simulink model "SistemaPF"  (R2024b)
settings: Solver=VariableStepAuto  StartTime=0.0  StopTime=10  RelTol=1e-3
libraries: slpidlib x1
settings Model: Creator=user
settings DataIOCC: TimeSaveName=t
settings DebuggingCC: UnconnectedInputMsg=warning  UnconnectedOutputMsg=warning  UnconnectedLineMsg=warning
settings ModelReferenceCC: EnableRefExpFcnMdlSchedulingChecks=on
settings RTWCC: GPUComputeCapability=3.5  DLArmComputeVersion=19.05

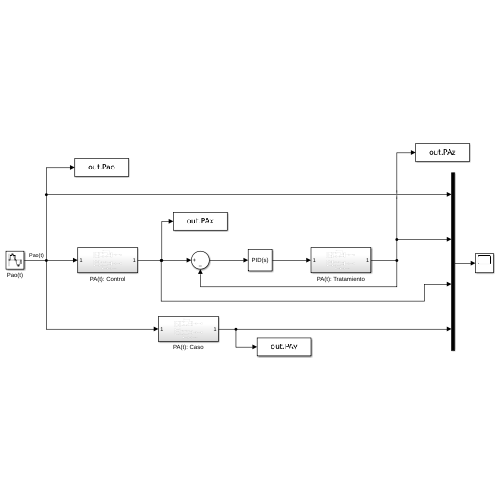
[thumbnail: Simulink's stored preview of the top-level diagram]
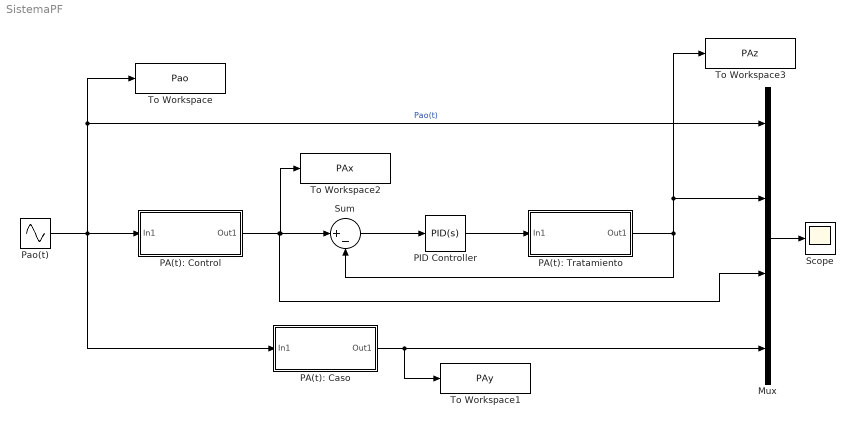
== system SistemaPF ==
  Mux : Mux
  PA(t): Caso : Subsystem
  PA(t): Control : Subsystem
  PA(t): Tratamiento : Subsystem
  PID Controller : slpidlib/PID Controller  Controller=PID  Form=Parallel  TimeDomain=Continuous-time  UseExternalTs=off  SampleTime=-1  IntegratorMethod=Forward Euler  FilterMethod=Forward Euler  ControllerParametersSource=internal  P=10.7123  I=13.7603  UseKiTs=off  D=1.4435  UseExternalDerivativeSource=off  N=651.125593180184  UseFilter=on  TunerSelectOption=Transfer Function Based (PID Tuner App)  InitialConditionSource=internal  InitialConditionForIntegrator=0  InitialConditionForFilter=0  DifferentiatorICPrevScaledInput=0  ExternalReset=none  TrackingMode=off  Kt=1  LimitOutput=off  SatLimitsSource=internal  UpperSaturationLimit=inf  LowerSaturationLimit=-inf  LinearizeAsGain=on  AntiWindupMode=none  Kb=1  LimitIntegrator=off  UpperIntegratorSaturationLimit=inf  LowerIntegratorSaturationLimit=-inf  POutMin=[]  POutMax=[]  IOutMin=[]  IOutMax=[]  DOutMin=[]  DOutMax=[]  NOutMin=[]  NOutMax=[]  SumOutMin=[]  SumOutMax=[]  SaturationOutMin=[]  SaturationOutMax=[]  PParamMin=[]  PParamMax=[]  IParamMin=[]  IParamMax=[]  DParamMin=[]  DParamMax=[]  NParamMin=[]  NParamMax=[]  KbParamMin=[]  KbParamMax=[]  KtParamMin=[]  KtParamMax=[]  KbOutMin=[]  KbOutMax=[]  KtOutMin=[]  KtOutMax=[]  IntegratorOutMin=[]  IntegratorOutMax=[]  FilterOutMin=[]  FilterOutMax=[]  SumI1OutMin=[]  SumI1OutMax=[]  SumI2OutMin=[]  SumI2OutMax=[]  SumI3OutMin=[]  SumI3OutMax=[]  SumI4OutMin=[]  SumI4OutMax=[]  SumDOutMin=[]  SumDOutMax=[]  DifferentiatorOutMin=[]  DifferentiatorOutMax=[]  FilterDiffOutCoefMin=[]  FilterDiffOutCoefMax=[]  ReciprocalOutMin=[]  ReciprocalOutMax=[]  SumDenOutMin=[]  SumDenOutMax=[]  SumNumOutMin=[]  SumNumOutMax=[]  DivideOutMin=[]  DivideOutMax=[]  UdiffTsProdOutMin=[]  UdiffTsProdOutMax=[]  NTsProdOutMin=[]  NTsProdOutMax=[]  UintegralTsProdOutMin=[]  UintegralTsProdOutMax=[]  UngainTsProdOutMin=[]  UngainTsProdOutMax=[]  ClampingZeroOutDataTypeStr=Inherit: Inherit via back propagation  ClampingZeroOutMin=[]  ClampingZeroOutMax=[]  FilterDenConstantOutDataTypeStr=Inherit: Inherit via back propagation  FilterDenConstantOutMin=[]  FilterDenConstantOutMax=[]  PCopyOutDataTypeStr=Inherit: Inherit via back propagation  PCopyOutMin=[]  PCopyOutMax=[]  NCopyOutDataTypeStr=Inherit: Inherit via back propagation  NCopyOutMin=[]  NCopyOutMax=[]  IntegratorContinuousStateAttributes=''  IntegratorStateMustResolveToSignalObject=off  IntegratorRTWStateStorageClass=Auto  FilterContinuousStateAttributes=''  FilterStateMustResolveToSignalObject=off  FilterRTWStateStorageClass=Auto  ParallelPVariant=InternalParameters  IdealPVariant=Disabled  IVariant=InternalParameters  DVariant=InternalParameters  IntegratorVariant=Continuous  SatVariant=Disabled  AWVariant=Passthrough  PCopyVariant=Disabled  TRVariant=Disabled  FdbkBlocksVariant=Forward  IdealPFdbkVariant=Disabled  SatFdbkVariant=Disabled  DerivativeFilterVariant=ContFilter  NVariant=InternalParameters  NCopyVariant=Disabled  FilterICVariant=InternalICsFilter  IntegratorICVariant=InternalICs  ExternalResetVariant=Disabled  TRSumVariant=Passthrough  SumFdbkVariant=Disabled  SumVariant=Sum_PID  TsampFilterVariant=InternalTs  TsampNgainVariant=Passthrough  TsampIntegralVariant=Disabled_SignalSpec  ExternalSaturationOutDataTypeStr=Inherit: Same as second input  DerivativeSourceVariant=ErrorSignal  PreIntVariant=InternalPreInt
  Pao(t) : Sin  Frequency=pi/2  SampleTime=0.001
  Scope : Scope
  Sum : Sum  Inputs=|+-
  To Workspace : ToWorkspace  VariableName=Pao  SampleTime=-1
  To Workspace1 : ToWorkspace  VariableName=PAy  SampleTime=-1
  To Workspace2 : ToWorkspace  VariableName=PAx  SampleTime=-1
  To Workspace3 : ToWorkspace  VariableName=PAz  SampleTime=-1
  wires:
  Sum/1 -> PID Controller/1
  Mux/1 -> Scope/1
  PA(t): Tratamiento/1(Out1) -> Sum/2, To Workspace3/1, Mux/2
  PA(t): Caso/1(Out1) -> To Workspace1/1, Mux/4
  PA(t): Control/1(Out1) -> Mux/3, To Workspace2/1, Sum/1
  PID Controller/1 -> PA(t): Tratamiento/1(In1)
  Pao(t)/1 -> PA(t): Caso/1(In1), To Workspace/1, Mux/1, PA(t): Control/1(In1)  "Pao(t)"

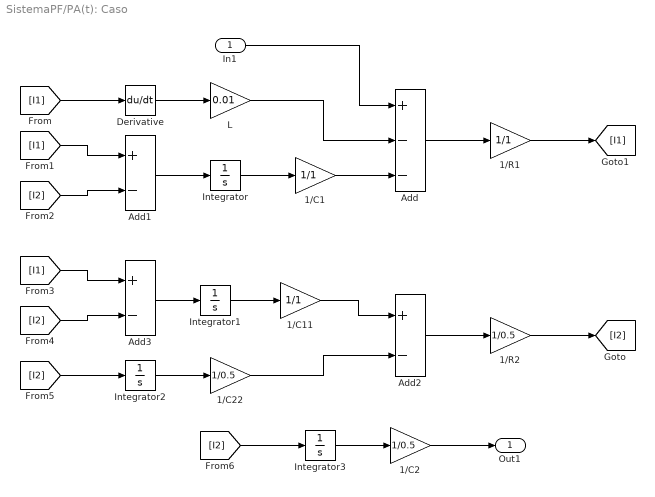
== system SistemaPF/PA(t): Caso ==
  In1 : Inport
  1/C1 : Gain  Gain=1/1
  1/C11 : Gain  Gain=1/1
  1/C2 : Gain  Gain=1/0.5
  1/C22 : Gain  Gain=1/0.5
  1/R1 : Gain  Gain=1/1
  1/R2 : Gain  Gain=1/0.5
  Add : Sum  Inputs=+--
  Add1 : Sum  Inputs=+-
  Add2 : Sum  Inputs=+-
  Add3 : Sum  Inputs=+-
  Derivative : Derivative
  Integrator{,1..3} (4 alike) : Integrator
  L : Gain  Gain=0.01
  Out1 : Outport
  wires:
  [I1] -> Derivative/1
  Derivative/1 -> L/1
  [I1] -> Add1/1
  [I2] -> Add1/2
  Add2/1 -> 1/R2/1
  1/R2/1 -> [I2]
  [I2] -> Add3/2
  [I1] -> Add3/1
  1/C11/1 -> Add2/1
  Add1/1 -> Integrator/1
  Integrator/1 -> 1/C1/1
  Add3/1 -> Integrator1/1
  Integrator1/1 -> 1/C11/1
  [I2] -> Integrator2/1
  Integrator2/1 -> 1/C22/1
  1/C22/1 -> Add2/2
  [I2] -> Integrator3/1
  Integrator3/1 -> 1/C2/1
  1/C2/1 -> Out1/1
  1/C1/1 -> Add/3
  L/1 -> Add/2
  In1/1 -> Add/1
  Add/1 -> 1/R1/1
  1/R1/1 -> [I1]

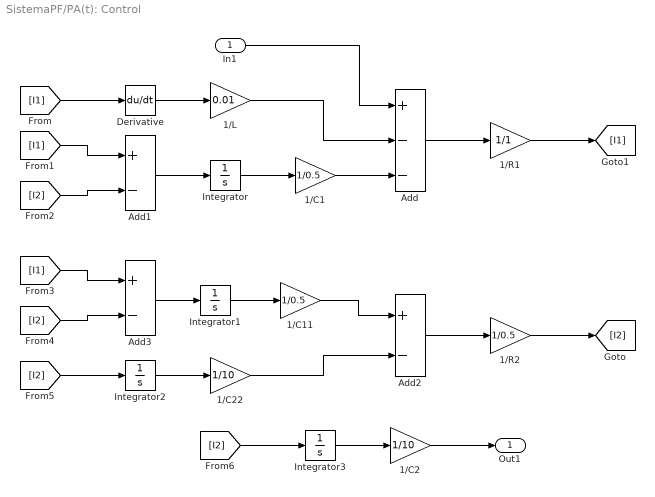
== system SistemaPF/PA(t): Control ==
  In1 : Inport
  1/C1 : Gain  Gain=1/0.5
  1/C11 : Gain  Gain=1/0.5
  1/C2 : Gain  Gain=1/10
  1/C22 : Gain  Gain=1/10
  1/L : Gain  Gain=0.01
  1/R1 : Gain  Gain=1/1
  1/R2 : Gain  Gain=1/0.5
  Add : Sum  Inputs=+--
  Add1 : Sum  Inputs=+-
  Add2 : Sum  Inputs=+-
  Add3 : Sum  Inputs=+-
  Derivative : Derivative
  Integrator{,1..3} (4 alike) : Integrator
  Out1 : Outport
  wires:
  [I1] -> Derivative/1
  Derivative/1 -> 1/L/1
  [I1] -> Add1/1
  [I2] -> Add1/2
  Add2/1 -> 1/R2/1
  1/R2/1 -> [I2]
  [I2] -> Add3/2
  [I1] -> Add3/1
  1/C11/1 -> Add2/1
  Add1/1 -> Integrator/1
  Integrator/1 -> 1/C1/1
  Add3/1 -> Integrator1/1
  Integrator1/1 -> 1/C11/1
  [I2] -> Integrator2/1
  Integrator2/1 -> 1/C22/1
  1/C22/1 -> Add2/2
  [I2] -> Integrator3/1
  Integrator3/1 -> 1/C2/1
  1/C2/1 -> Out1/1
  1/C1/1 -> Add/3
  1/L/1 -> Add/2
  In1/1 -> Add/1
  Add/1 -> 1/R1/1
  1/R1/1 -> [I1]

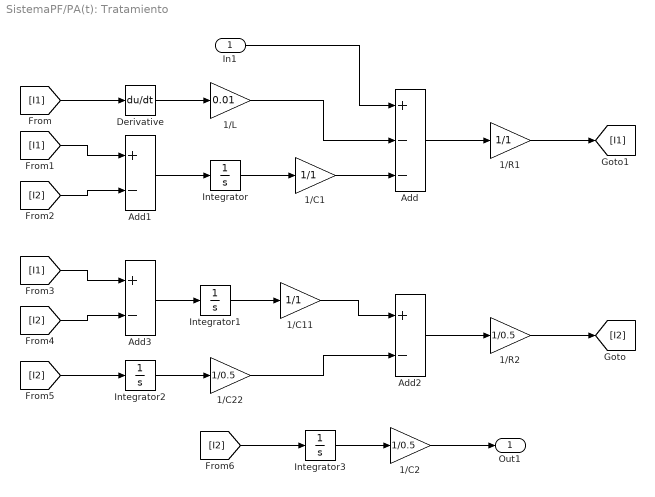
== system SistemaPF/PA(t): Tratamiento ==
  In1 : Inport
  1/C1 : Gain  Gain=1/1
  1/C11 : Gain  Gain=1/1
  1/C2 : Gain  Gain=1/0.5
  1/C22 : Gain  Gain=1/0.5
  1/L : Gain  Gain=0.01
  1/R1 : Gain  Gain=1/1
  1/R2 : Gain  Gain=1/0.5
  Add : Sum  Inputs=+--
  Add1 : Sum  Inputs=+-
  Add2 : Sum  Inputs=+-
  Add3 : Sum  Inputs=+-
  Derivative : Derivative
  Integrator{,1..3} (4 alike) : Integrator
  Out1 : Outport
  wires:
  [I1] -> Derivative/1
  Derivative/1 -> 1/L/1
  [I1] -> Add1/1
  [I2] -> Add1/2
  Add2/1 -> 1/R2/1
  1/R2/1 -> [I2]
  [I2] -> Add3/2
  [I1] -> Add3/1
  1/C11/1 -> Add2/1
  Add1/1 -> Integrator/1
  Integrator/1 -> 1/C1/1
  Add3/1 -> Integrator1/1
  Integrator1/1 -> 1/C11/1
  [I2] -> Integrator2/1
  Integrator2/1 -> 1/C22/1
  1/C22/1 -> Add2/2
  [I2] -> Integrator3/1
  Integrator3/1 -> 1/C2/1
  1/C2/1 -> Out1/1
  1/C1/1 -> Add/3
  1/L/1 -> Add/2
  In1/1 -> Add/1
  Add/1 -> 1/R1/1
  1/R1/1 -> [I1]
